simulink model "Spring_Mass_System"  (R2024a)
settings: Solver=VariableStepAuto  StartTime=0.0  StopTime=10.0  RelTol=1e-3
settings Model: Creator=Lenovo  LastModifiedBy=Lenovo

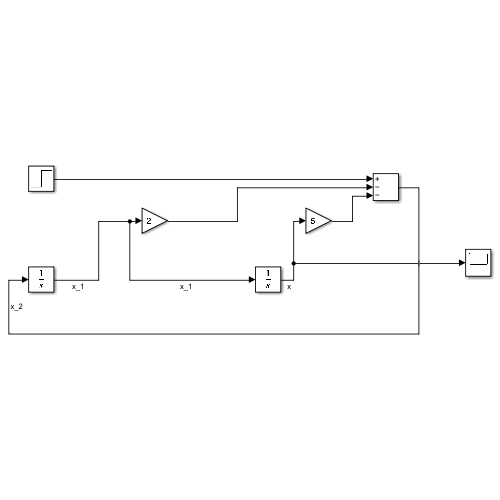
[thumbnail: Simulink's stored preview of the top-level diagram]
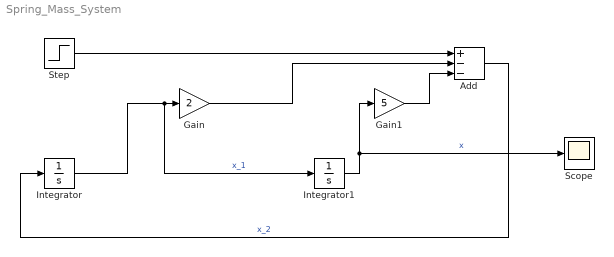
== system Spring_Mass_System ==
  Add : Sum  Inputs=+--
  Gain : Gain  Gain=2
  Gain1 : Gain  Gain=5
  Integrator : Integrator
  Integrator1 : Integrator
  Scope : Scope
  Step : Step  Time=0  SampleTime=0
  wires:
  Add/1 -> Integrator/1  "x_2"
  Integrator1/1 -> Gain1/1, Scope/1  "x"
  Step/1 -> Add/1
  Integrator/1 -> Integrator1/1, Gain/1  "x_1"
  Gain/1 -> Add/2
  Gain1/1 -> Add/3
